simulink model "InverseDynamicsTest"  (R2021b)
settings: Solver=FixedStepAuto  StartTime=0.0  StopTime=5  FixedStep=Ts  RelTol=1e-3
values from neighbouring files (symbols this model uses):
  alphas_m = 25.0 * ones(1,dh.dof)    [setup_teleop.m]
  gravity = [0 0 9.81]'    [setup_robot.m]
  lambdas_m = 7.5 * ones(1,dh.dof)    [setup_teleop.m]
  zdq_A = [1 3*wc 3*wc^2 wc^3]    [setup_teleop.m]
  zdq_B = [0 0 0 wc^3]    [setup_teleop.m]
undefined symbols (not defined in the file or in its folder): conf, dh, x0
libraries: simulink x2, robotcorelib x1, vrlib x1
settings Model: Creator=eros  LastModifiedBy=Sebastiano
settings SolverCC: AlgebraicLoopSolver=TrustRegion
settings DebuggingCC: SFMachineParentedDataDiag=warning

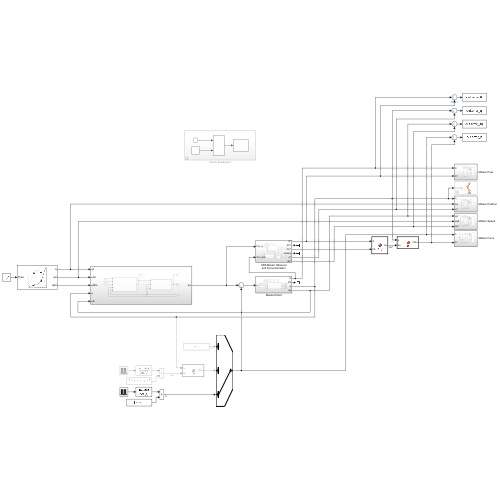
[thumbnail: Simulink's stored preview of the top-level diagram]
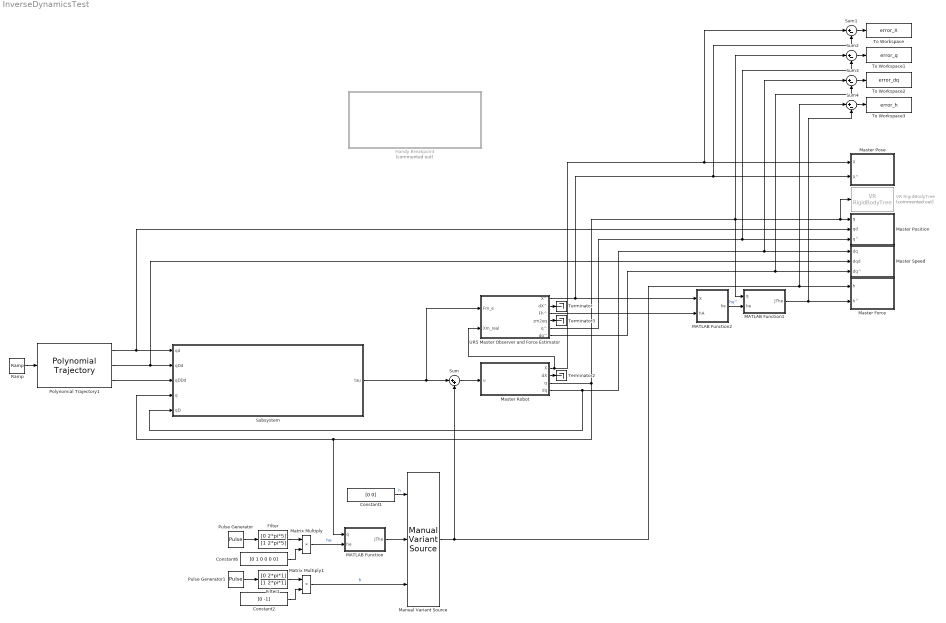
== system InverseDynamicsTest ==
  Constant1 : Constant  Value=[0 0]
  Constant2 : Constant  Value=[0 -1]
  Constant6 : Constant  Value=[0 1 0 0 0 0]
  Filter : TransferFcn  Numerator=[0 2*pi*5]  Denominator=[1 2*pi*5]
  Filter1 : TransferFcn  Numerator=[0 2*pi*1]  Denominator=[1 2*pi*1]
  Handy Breakpoint : Subsystem  Commented=on
  MATLAB Function : MATLAB Function  TreatAsAtomicUnit=on
  MATLAB Function1 : MATLAB Function  TreatAsAtomicUnit=on
  MATLAB Function2 : MATLAB Function  TreatAsAtomicUnit=on
  Manual Variant Source : simulink/Signal Routing/Manual Variant Source  NumChoices=3  LabelModeActiveChoice=V_3
  Master Force : Subsystem
  Master Pose : Subsystem
  Master Position : Subsystem
  Master Robot : Subsystem
  Master Speed : Subsystem
  Matrix Multiply : Product
  Matrix Multiply1 : Product
  Polynomial Trajectory1 : robotcorelib/Polynomial Trajectory  WaypointSource=Internal  Waypoints=[conf.init.q0 conf.init.q0]  TimePoints=[ 0, 5]  TimeInterval=[ 1, 4 ]  Method=Cubic Polynomial  ParameterSource=Internal  VelocityBoundaryCondition=zeros( dh.dof, 2 )  AccelerationBoundaryCondition=zeros( 2, 5 )  SimulateUsing=Code generation
  Pulse Generator : DiscretePulseGenerator  PulseType=Time based  Amplitude=25  Period=3  PulseWidth=50  PhaseDelay=0.5
  Pulse Generator1 : DiscretePulseGenerator  PulseType=Time based  Amplitude=25  Period=3  PulseWidth=50  PhaseDelay=0.5
  Ramp : simulink/Sources/Ramp  slope=1  start=0  InitialOutput=0
  Subsystem : Subsystem
  Sum : Sum  Inputs=|++
  Sum{1..4} (4 alike) : Sum  Inputs=|+-
  Terminator : Terminator
  Terminator2 : Terminator
  Terminator3 : Terminator
  To Workspace : ToWorkspace  VariableName=error_X  SaveFormat=Timeseries  SampleTime=-1
  To Workspace1 : ToWorkspace  VariableName=error_q  SaveFormat=Timeseries  SampleTime=-1
  To Workspace2 : ToWorkspace  VariableName=error_dq  SaveFormat=Timeseries  SampleTime=-1
  To Workspace3 : ToWorkspace  VariableName=error_h  SaveFormat=Timeseries  SampleTime=-1
  UR5 Master Observer and Force Estimator : Subsystem
  VR RigidBodyTree : vrlib/VR RigidBodyTree  Commented=on  RBT=UR5_robot  useRBT=off  Ts=0.02  ForceViewerOpen=off
      settings: SourceProductBaseCode=SL
  wires:
  Master Robot/4(dq) -> Sum3/1, Master Speed/1(dq), Subsystem/5(qD)
  Polynomial Trajectory1/1 -> Master Position/2(qd), Subsystem/1(qd)
  Polynomial Trajectory1/2 -> Master Speed/2(dqd), Subsystem/2(qDd)
  Ramp/1 -> Polynomial Trajectory1/1
  Sum/1 -> Master Robot/1(u)
  Manual Variant Source/1 -> Master Force/1(h), Sum4/1, Sum/2
  Pulse Generator/1 -> Filter/1
  Constant6/1 -> Matrix Multiply/2
  Matrix Multiply/1 -> MATLAB Function/2(he)  "he"
  Filter/1 -> Matrix Multiply/1
  UR5 Master Observer and Force Estimator/5(q^) -> Master Position/3(q^), Sum2/2
  UR5 Master Observer and Force Estimator/3(Fh^) -> MATLAB Function2/2(hA)
  UR5 Master Observer and Force Estimator/6(dq^) -> Master Speed/3(dq^), Sum3/2
  Master Robot/1(X) -> Master Pose/1(X), Sum1/1, UR5 Master Observer and Force Estimator/2(Xm_real)
  Master Robot/2(dX) -> Terminator2/1
  UR5 Master Observer and Force Estimator/4(zm2eq) -> Terminator3/1
  UR5 Master Observer and Force Estimator/2(dX^) -> Terminator/1
  UR5 Master Observer and Force Estimator/1(X^) -> Master Pose/2(X^), Sum1/2, MATLAB Function2/1(X)
  Constant1/1 -> Manual Variant Source/1  "h"
  MATLAB Function2/1(he) -> MATLAB Function1/2(he)  "he^"
  Master Robot/3(q) -> VR RigidBodyTree/1, Master Position/1(q), MATLAB Function1/1(q), Sum2/1, Subsystem/4(q), MATLAB Function/1(q)
  MATLAB Function1/1(JThe) -> Master Force/2(h^), Sum4/2
  MATLAB Function/1(JThe) -> Manual Variant Source/2
  Matrix Multiply1/1 -> Manual Variant Source/3  "h"
  Constant2/1 -> Matrix Multiply1/2
  Filter1/1 -> Matrix Multiply1/1
  Pulse Generator1/1 -> Filter1/1
  Sum1/1 -> To Workspace/1
  Sum2/1 -> To Workspace1/1
  Sum3/1 -> To Workspace2/1
  Sum4/1 -> To Workspace3/1
  Subsystem/1(tau) -> Sum/1, UR5 Master Observer and Force Estimator/1(Fm_e)
  Polynomial Trajectory1/3 -> Subsystem/3(qDDd)

== system InverseDynamicsTest/Handy Breakpoint ==
  Assertion : Assertion  AssertionFailFcn=set_param(bdroot,'SimulationCommand','pause')  StopWhenAssertionFail=off
  Clock : Clock
  Constant : Constant  Value=0.5
  Relational Operator : RelationalOperator  Operator=<  OutDataTypeStr=boolean  RndMeth=Simplest
  wires:
  Relational Operator/1 -> Assertion/1
  Constant/1 -> Relational Operator/2
  Clock/1 -> Relational Operator/1

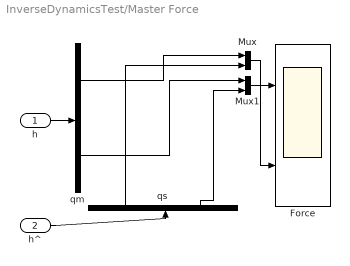
== system InverseDynamicsTest/Master Force ==
  h : Inport
  h^ : Inport  Port=2
  Force : Scope  NumInputPorts=2
  Mux : Mux  Inputs=2
  Mux1 : Mux  Inputs=2
  qm : Demux  Outputs=dh.dof
  qs : Demux  Outputs=dh.dof
  wires:
  h/1 -> qm/1
  h^/1 -> qs/1
  qm/1 -> Mux/1
  qs/1 -> Mux/2
  qm/2 -> Mux1/1
  qs/2 -> Mux1/2
  Mux/1 -> Force/1
  Mux1/1 -> Force/2

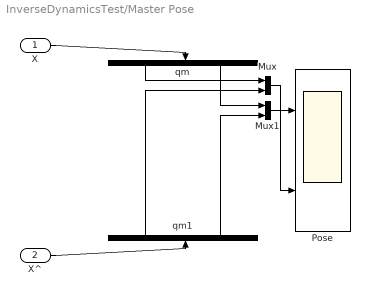
== system InverseDynamicsTest/Master Pose ==
  X : Inport
  X^ : Inport  Port=2
  Mux : Mux  Inputs=2
  Mux1 : Mux  Inputs=2
  Pose : Scope  NumInputPorts=2
  qm : Demux  Outputs=dh.dof
  qm1 : Demux  Outputs=dh.dof
  wires:
  X/1 -> qm/1
  qm/1 -> Mux/1
  qm/2 -> Mux1/1
  Mux/1 -> Pose/1
  Mux1/1 -> Pose/2
  qm1/2 -> Mux1/2
  X^/1 -> qm1/1
  qm1/1 -> Mux/2

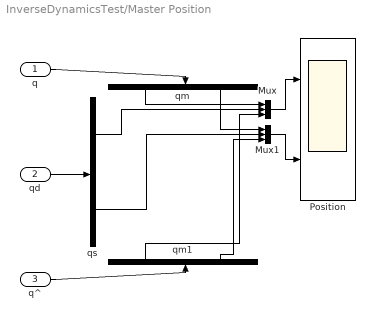
== system InverseDynamicsTest/Master Position ==
  q : Inport
  qd : Inport  Port=2
  q^ : Inport  Port=3
  Mux : Mux  Inputs=3
  Mux1 : Mux  Inputs=3
  Position : Scope  NumInputPorts=2
  qm : Demux  Outputs=dh.dof
  qm1 : Demux  Outputs=dh.dof
  qs : Demux  Outputs=dh.dof
  wires:
  q/1 -> qm/1
  qd/1 -> qs/1
  qm/1 -> Mux/1
  qs/1 -> Mux/2
  qm/2 -> Mux1/1
  qs/2 -> Mux1/2
  Mux/1 -> Position/1
  Mux1/1 -> Position/2
  qm1/2 -> Mux1/3
  q^/1 -> qm1/1
  qm1/1 -> Mux/3

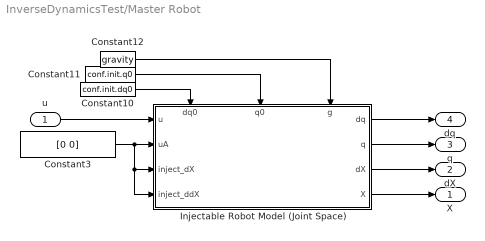
== system InverseDynamicsTest/Master Robot ==
  u : Inport
  Constant10 : Constant  Value=conf.init.dq0
  Constant11 : Constant  Value=conf.init.q0
  Constant12 : Constant  Value=gravity
  Constant3 : Constant  Value=[0 0]
  Injectable Robot Model (Joint Space) : Subsystem
      settings: PortSchema="{\"entries\":[{\"content\":{\"sides\":[{\"content\":{\"connectorIds\":[\"In1\",\"In2\",\"In3\",\"In4\"]},\"type\":\"ConnectorPlacement.EquallySpacedRectSide\",\"uuid\":\"a8701c64-329e-4144-b882-ecf5d621aff2\"},{\"content\":{\"connectorIds\":[\"Out1\",\"Out2\",\"Out3\",\"Out4\"],\"side\":\"RIGHT\"},\"type\":\"ConnectorPlacement.EquallySpacedRectSide\",\"uuid\":\"4e168703-1cb9-438c-bc6b-9b2d7fbb809e\"},{\"content\":{\"connectorIds\":[\"In5\",\"In6\",\"In7\"],\"side\":\"TOP\"},\"type\":\"ConnectorPlacement.EquallySpacedRectSide\",\"uuid\":\"8fbcb29e-7fab-4224-b4ad-ee01c13d675a\"}]},\"type\":\"ConnectorPlacement.EquallySpacedConnector\",\"uuid\":\"fa721fab-1ce6-4fdf-95fa-8ada3ed2d65c\"}],\"packageUris\":[\"http://schema.mathworks.com/mf0/Connector/R2020b\"],\"version\":\"1.0\"}"
  X : Outport
  dX : Outport  Port=2
  q : Outport  Port=3
  dq : Outport  Port=4
  wires:
  Constant10/1 -> Injectable Robot Model (Joint Space)/5(dq0)
  Constant3/1 -> Injectable Robot Model (Joint Space)/4(inject_ddX), Injectable Robot Model (Joint Space)/3(inject_dX), Injectable Robot Model (Joint Space)/2(uA)
  Constant11/1 -> Injectable Robot Model (Joint Space)/6(q0)
  Injectable Robot Model (Joint Space)/2(q) -> q/1
  Injectable Robot Model (Joint Space)/3(dX) -> dX/1
  Constant12/1 -> Injectable Robot Model (Joint Space)/7(g)
  Injectable Robot Model (Joint Space)/4(X) -> X/1
  Injectable Robot Model (Joint Space)/1(dq) -> dq/1
  u/1 -> Injectable Robot Model (Joint Space)/1(u)

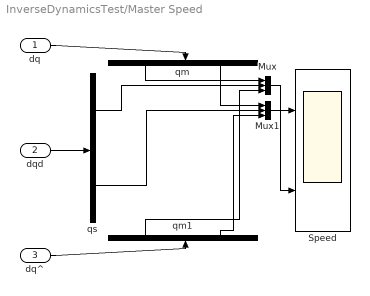
== system InverseDynamicsTest/Master Speed ==
  dq : Inport
  dqd : Inport  Port=2
  dq^ : Inport  Port=3
  Mux : Mux  Inputs=3
  Mux1 : Mux  Inputs=3
  Speed : Scope  NumInputPorts=2
  qm : Demux  Outputs=dh.dof
  qm1 : Demux  Outputs=dh.dof
  qs : Demux  Outputs=dh.dof
  wires:
  dq/1 -> qm/1
  dqd/1 -> qs/1
  qm/1 -> Mux/1
  qs/1 -> Mux/2
  qm/2 -> Mux1/1
  qs/2 -> Mux1/2
  Mux/1 -> Speed/1
  Mux1/1 -> Speed/2
  qm1/2 -> Mux1/3
  dq^/1 -> qm1/1
  qm1/1 -> Mux/3

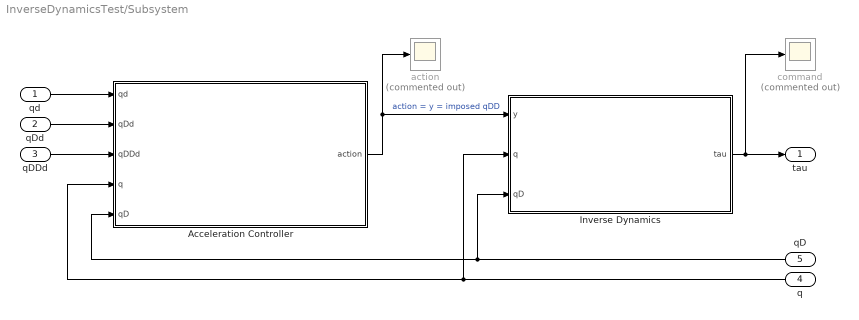
== system InverseDynamicsTest/Subsystem ==
  qd : Inport
  qDd : Inport  Port=2
  qDDd : Inport  Port=3
  q : Inport  Port=4
  qD : Inport  Port=5
  Acceleration Controller : Subsystem
  Inverse Dynamics : Subsystem
  action : Scope  Commented=on
  command : Scope  Commented=on
  tau : Outport
  wires:
  qD/1 -> Acceleration Controller/5(qD), Inverse Dynamics/3(qD)
  qd/1 -> Acceleration Controller/1(qd)
  q/1 -> Inverse Dynamics/2(q), Acceleration Controller/4(q)
  Inverse Dynamics/1(tau) -> tau/1, command/1
  qDDd/1 -> Acceleration Controller/3(qDDd)
  qDd/1 -> Acceleration Controller/2(qDd)
  Acceleration Controller/1(action) -> Inverse Dynamics/1(y), action/1  "action = y = imposed qDD"

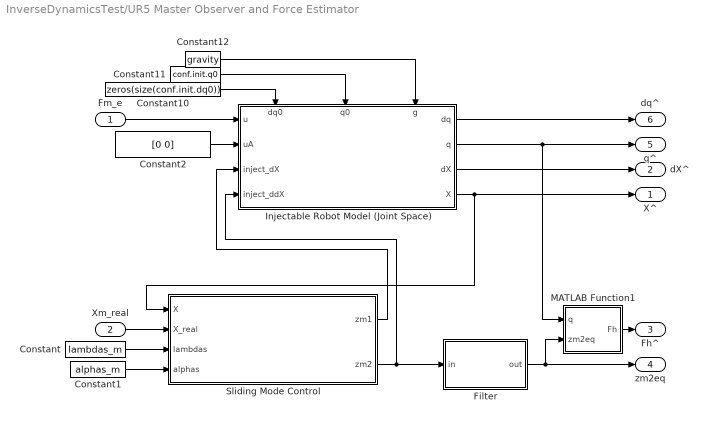
== system InverseDynamicsTest/UR5 Master Observer and Force Estimator ==
  Fm_e : Inport
  Xm_real : Inport  Port=2
  Constant : Constant  Value=lambdas_m
  Constant1 : Constant  Value=alphas_m
  Constant10 : Constant  Value=zeros(size(conf.init.dq0))
  Constant11 : Constant  Value=conf.init.q0
  Constant12 : Constant  Value=gravity
  Constant2 : Constant  Value=[0 0]
  Filter : Subsystem
  Injectable Robot Model (Joint Space) : Subsystem
      settings: PortSchema="{\"entries\":[{\"content\":{\"sides\":[{\"content\":{\"connectorIds\":[\"In1\",\"In2\",\"In3\",\"In4\"]},\"type\":\"ConnectorPlacement.EquallySpacedRectSide\",\"uuid\":\"a8701c64-329e-4144-b882-ecf5d621aff2\"},{\"content\":{\"connectorIds\":[\"Out1\",\"Out2\",\"Out3\",\"Out4\"],\"side\":\"RIGHT\"},\"type\":\"ConnectorPlacement.EquallySpacedRectSide\",\"uuid\":\"4e168703-1cb9-438c-bc6b-9b2d7fbb809e\"},{\"content\":{\"connectorIds\":[\"In5\",\"In6\",\"In7\"],\"side\":\"TOP\"},\"type\":\"ConnectorPlacement.EquallySpacedRectSide\",\"uuid\":\"8fbcb29e-7fab-4224-b4ad-ee01c13d675a\"}]},\"type\":\"ConnectorPlacement.EquallySpacedConnector\",\"uuid\":\"fa721fab-1ce6-4fdf-95fa-8ada3ed2d65c\"}],\"packageUris\":[\"http://schema.mathworks.com/mf0/Connector/R2020b\"],\"version\":\"1.0\"}"
  MATLAB Function1 : MATLAB Function  TreatAsAtomicUnit=on
  Sliding Mode Control : Subsystem
  X^ : Outport
  dX^ : Outport  Port=2
  Fh^ : Outport  Port=3
  zm2eq : Outport  Port=4
  q^ : Outport  Port=5
  dq^ : Outport  Port=6
  wires:
  Filter/1(out) -> MATLAB Function1/2(zm2eq), zm2eq/1
  Sliding Mode Control/1(zm1) -> Injectable Robot Model (Joint Space)/3(inject_dX)
  Sliding Mode Control/2(zm2) -> Injectable Robot Model (Joint Space)/4(inject_ddX), Filter/1(in)
  Constant1/1 -> Sliding Mode Control/4(alphas)
  Constant/1 -> Sliding Mode Control/3(lambdas)
  Xm_real/1 -> Sliding Mode Control/2(X_real)
  Injectable Robot Model (Joint Space)/4(X) -> X^/1, Sliding Mode Control/1(X)
  Injectable Robot Model (Joint Space)/3(dX) -> dX^/1
  Constant11/1 -> Injectable Robot Model (Joint Space)/6(q0)
  Fm_e/1 -> Injectable Robot Model (Joint Space)/1(u)
  Constant10/1 -> Injectable Robot Model (Joint Space)/5(dq0)
  Injectable Robot Model (Joint Space)/1(dq) -> dq^/1
  Constant12/1 -> Injectable Robot Model (Joint Space)/7(g)
  Injectable Robot Model (Joint Space)/2(q) -> MATLAB Function1/1(q), q^/1
  MATLAB Function1/1(Fh) -> Fh^/1
  Constant2/1 -> Injectable Robot Model (Joint Space)/2(uA)

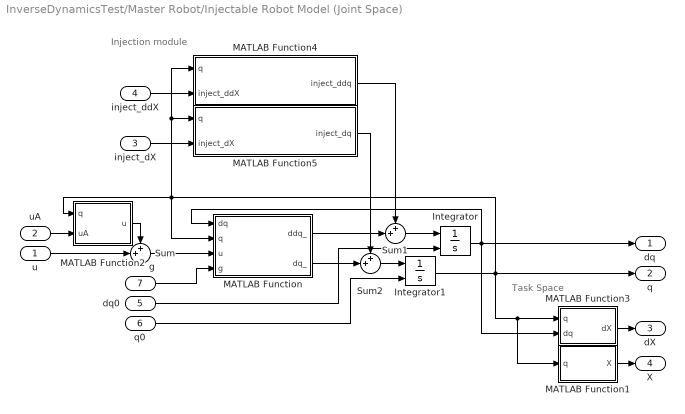
== system InverseDynamicsTest/Master Robot/Injectable Robot Model (Joint Space) ==
  note: Injection module
  note: Task Space
  u : Inport
  uA : Inport  Port=2
  inject_dX : Inport  Port=3
  inject_ddX : Inport  Port=4
  dq0 : Inport  Port=5
  q0 : Inport  Port=6
  g : Inport  Port=7
  Integrator : Integrator  InitialConditionSource=external  InitialCondition=x0
  Integrator1 : Integrator  InitialConditionSource=external  InitialCondition=x0
  MATLAB Function : MATLAB Function  TreatAsAtomicUnit=on
  MATLAB Function1 : MATLAB Function  TreatAsAtomicUnit=on
  MATLAB Function2 : MATLAB Function  TreatAsAtomicUnit=on
  MATLAB Function3 : MATLAB Function  TreatAsAtomicUnit=on
  MATLAB Function4 : MATLAB Function  TreatAsAtomicUnit=on
  MATLAB Function5 : MATLAB Function  TreatAsAtomicUnit=on
  Sum : Sum  Inputs=++|
  Sum1 : Sum  Inputs=++|
  Sum2 : Sum  Inputs=++|
  dq : Outport
  q : Outport  Port=2
  dX : Outport  Port=3
  X : Outport  Port=4
  wires:
  g/1 -> MATLAB Function/4(g)
  u/1 -> Sum/2
  dq0/1 -> Integrator/2
  Integrator1/1 -> q/1, MATLAB Function1/1(q), MATLAB Function3/1(q), MATLAB Function/2(q), MATLAB Function4/1(q), MATLAB Function5/1(q), MATLAB Function2/1(q)
  uA/1 -> MATLAB Function2/2(uA)
  MATLAB Function1/1(X) -> X/1
  Integrator/1 -> dq/1, MATLAB Function3/2(dq), MATLAB Function/1(dq)
  MATLAB Function3/1(dX) -> dX/1
  MATLAB Function2/1(u) -> Sum/1
  Sum/1 -> MATLAB Function/3(u)
  MATLAB Function/1(ddq_) -> Sum1/2
  q0/1 -> Integrator1/2
  Sum1/1 -> Integrator/1
  MATLAB Function/2(dq_) -> Sum2/2
  Sum2/1 -> Integrator1/1
  inject_ddX/1 -> MATLAB Function4/2(inject_ddX)
  inject_dX/1 -> MATLAB Function5/2(inject_dX)
  MATLAB Function4/1(inject_ddq) -> Sum1/1
  MATLAB Function5/1(inject_dq) -> Sum2/1

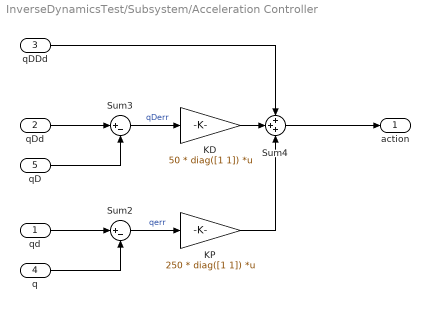
== system InverseDynamicsTest/Subsystem/Acceleration Controller ==
  qd : Inport
  qDd : Inport  Port=2
  qDDd : Inport  Port=3
  q : Inport  Port=4
  qD : Inport  Port=5
  KD : Gain  Gain=50 * diag([1 1])  Multiplication=Matrix(K*u) (u vector)
  KP : Gain  Gain=250 * diag([1 1])  Multiplication=Matrix(K*u) (u vector)
  Sum2 : Sum  Inputs=|+-
  Sum3 : Sum  Inputs=|+-
  Sum4 : Sum  Inputs=+++
  action : Outport
  wires:
  qDd/1 -> Sum3/1
  KD/1 -> Sum4/2
  KP/1 -> Sum4/3
  qD/1 -> Sum3/2
  Sum3/1 -> KD/1  "qDerr"
  Sum4/1 -> action/1
  Sum2/1 -> KP/1  "qerr"
  qd/1 -> Sum2/1
  qDDd/1 -> Sum4/1
  q/1 -> Sum2/2

== system InverseDynamicsTest/Subsystem/Inverse Dynamics ==
  y : Inport
  q : Inport  Port=2
  qD : Inport  Port=3
  MATLAB Function : MATLAB Function  TreatAsAtomicUnit=on
  MATLAB Function1 : MATLAB Function  TreatAsAtomicUnit=on
  Sum1 : Sum  Inputs=++|
  tau : Outport
  wires:
  qD/1 -> MATLAB Function/2(qD)
  MATLAB Function/1(n) -> Sum1/1
  MATLAB Function1/1(taud) -> Sum1/2
  q/1 -> MATLAB Function1/1(q), MATLAB Function/1(q)
  y/1 -> MATLAB Function1/2(y)
  Sum1/1 -> tau/1  "tau"

== system InverseDynamicsTest/UR5 Master Observer and Force Estimator/Filter ==
  in : Inport
  Demux : Demux  Outputs=2
  Filter : TransferFcn  Numerator=zdq_B  Denominator=zdq_A
  Filter1 : TransferFcn  Numerator=zdq_B  Denominator=zdq_A
  Mux : Mux  Inputs=2
  out : Outport
  wires:
  Demux/2 -> Filter1/1
  Demux/1 -> Filter/1
  in/1 -> Demux/1
  Mux/1 -> out/1
  Filter/1 -> Mux/1
  Filter1/1 -> Mux/2

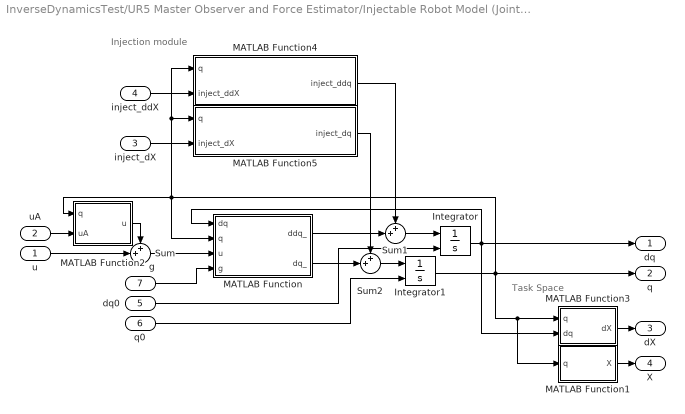
== system InverseDynamicsTest/UR5 Master Observer and Force Estimator/Injectable Robot Model (Joint Space) ==
  note: Injection module
  note: Task Space
  u : Inport
  uA : Inport  Port=2
  inject_dX : Inport  Port=3
  inject_ddX : Inport  Port=4
  dq0 : Inport  Port=5
  q0 : Inport  Port=6
  g : Inport  Port=7
  Integrator : Integrator  InitialConditionSource=external  InitialCondition=x0
  Integrator1 : Integrator  InitialConditionSource=external  InitialCondition=x0
  MATLAB Function : MATLAB Function  TreatAsAtomicUnit=on
  MATLAB Function1 : MATLAB Function  TreatAsAtomicUnit=on
  MATLAB Function2 : MATLAB Function  TreatAsAtomicUnit=on
  MATLAB Function3 : MATLAB Function  TreatAsAtomicUnit=on
  MATLAB Function4 : MATLAB Function  TreatAsAtomicUnit=on
  MATLAB Function5 : MATLAB Function  TreatAsAtomicUnit=on
  Sum : Sum  Inputs=++|
  Sum1 : Sum  Inputs=++|
  Sum2 : Sum  Inputs=++|
  dq : Outport
  q : Outport  Port=2
  dX : Outport  Port=3
  X : Outport  Port=4
  wires:
  g/1 -> MATLAB Function/4(g)
  u/1 -> Sum/2
  dq0/1 -> Integrator/2
  Integrator1/1 -> q/1, MATLAB Function1/1(q), MATLAB Function3/1(q), MATLAB Function/2(q), MATLAB Function4/1(q), MATLAB Function5/1(q), MATLAB Function2/1(q)
  uA/1 -> MATLAB Function2/2(uA)
  MATLAB Function1/1(X) -> X/1
  Integrator/1 -> dq/1, MATLAB Function3/2(dq), MATLAB Function/1(dq)
  MATLAB Function3/1(dX) -> dX/1
  MATLAB Function2/1(u) -> Sum/1
  Sum/1 -> MATLAB Function/3(u)
  MATLAB Function/1(ddq_) -> Sum1/2
  q0/1 -> Integrator1/2
  Sum1/1 -> Integrator/1
  MATLAB Function/2(dq_) -> Sum2/2
  Sum2/1 -> Integrator1/1
  inject_ddX/1 -> MATLAB Function4/2(inject_ddX)
  inject_dX/1 -> MATLAB Function5/2(inject_dX)
  MATLAB Function4/1(inject_ddq) -> Sum1/1
  MATLAB Function5/1(inject_dq) -> Sum2/1

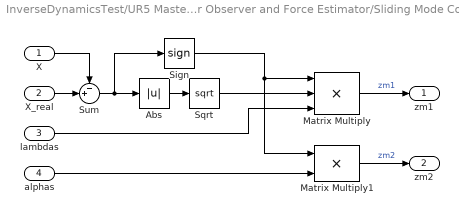
== system InverseDynamicsTest/UR5 Master Observer and Force Estimator/Sliding Mode Control ==
  X : Inport
  X_real : Inport  Port=2
  lambdas : Inport  Port=3
  alphas : Inport  Port=4
  Abs : Abs
  Matrix Multiply : Product  Inputs=***
  Matrix Multiply1 : Product
  Sign : Signum
  Sqrt : Sqrt  SaturateOnIntegerOverflow=on
  Sum : Sum  Inputs=-+|
  zm1 : Outport
  zm2 : Outport  Port=2
  wires:
  Sum/1 -> Sign/1, Abs/1
  Abs/1 -> Sqrt/1
  X/1 -> Sum/1
  lambdas/1 -> Matrix Multiply/3
  Sqrt/1 -> Matrix Multiply/2
  X_real/1 -> Sum/2
  Matrix Multiply/1 -> zm1/1  "zm1"
  Matrix Multiply1/1 -> zm2/1  "zm2"
  alphas/1 -> Matrix Multiply1/2
  Sign/1 -> Matrix Multiply/1, Matrix Multiply1/1

== matlab function InverseDynamicsTest/Subsystem/Inverse Dynamics/MATLAB Function ==
  data: q input; qD input; n output; dh parameter; gravity parameter
function n = n(q, qD, dh, gravity)

    C = C_rne(dh, q, qD);
    G = G_rne(dh, q, gravity);

    n = C * qD + G;

== matlab function InverseDynamicsTest/Master Robot/Injectable Robot Model (Joint Space)/MATLAB Function5 ==
  data: q input size=dh.dof; inject_dq output size=dh.dof; inject_dX input size=2; dh parameter
function inject_dq = get_inject_dq(q, inject_dX, dh)
    JA = JA_rne(dh, q);
    inject_dq = pinv(JA) * inject_dX;
end

== matlab function InverseDynamicsTest/Subsystem/Inverse Dynamics/MATLAB Function1 ==
  data: q input; taud output; y input; dh parameter
function taud = B(q, y, dh)

    B = B_rne(dh, q);

    taud = B*y;

== matlab function InverseDynamicsTest/UR5 Master Observer and Force Estimator/Injectable Robot Model (Joint Space)/MATLAB Function1 ==
  data: X output; q input; dh parameter
function X = K(q, dh)
    X = K_rne(dh, q);
end

== matlab function InverseDynamicsTest/MATLAB Function ==
  data: JThe output; q input; he input; dh parameter
function JThe = JT(q, he, dh)
    JThe = J_rne(dh, q)' * he;
end

== matlab function InverseDynamicsTest/UR5 Master Observer and Force Estimator/Injectable Robot Model (Joint Space)/MATLAB Function3 ==
  data: dh parameter; dX output; q input; dq input
function dX = JA(dh, q, dq)
    dX = JA_rne(dh, q)*dq;
end

== matlab function InverseDynamicsTest/UR5 Master Observer and Force Estimator/Injectable Robot Model (Joint Space)/MATLAB Function4 ==
  data: q input size=dh.dof; inject_ddq output size=dh.dof; inject_ddX input size=2; dh parameter
function inject_ddq = get_inject_ddq(q, inject_ddX, dh)
    JA = JA_rne(dh, q);
    inject_ddq = pinv(JA) * inject_ddX;
end

== matlab function InverseDynamicsTest/MATLAB Function1 ==
  data: JThe output; q input; he input; dh parameter
function JThe = JT(q, he, dh)
    JThe = J_rne(dh, q)' * he;
end

== matlab function InverseDynamicsTest/UR5 Master Observer and Force Estimator/Injectable Robot Model (Joint Space)/MATLAB Function5 ==
  data: q input size=dh.dof; inject_dq output size=dh.dof; inject_dX input size=2; dh parameter
function inject_dq = get_inject_dq(q, inject_dX, dh)
    JA = JA_rne(dh, q);
    inject_dq = pinv(JA) * inject_dX;
end

== matlab function InverseDynamicsTest/Master Robot/Injectable Robot Model (Joint Space)/MATLAB Function ==
  data ddq_ settings: updateMethod=SF_CONTINUOUS_TIME_DATA
  data dq_ settings: updateMethod=SF_CONTINUOUS_TIME_DATA
  data dq settings: updateMethod=SF_CONTINUOUS_TIME_DATA
  data q settings: updateMethod=SF_CONTINUOUS_TIME_DATA
  data u settings: updateMethod=SF_CONTINUOUS_TIME_DATA
  data: ddq_ output size=dh.dof; dq_ output size=dh.dof; dq input size=dh.dof; q input size=dh.dof; u input size=dh.dof; g input size=3; dh parameter
function [ddq_, dq_]  = RobotSystem(dq, q, u, g, dh)
    
    % compute dynamics
    B = B_rne(dh, q);
    C = C_rne(dh, q, dq);
    G = G_rne(dh, q, g);

    dq_ = dq(1:dh.dof);

    ddq = B \ (u - C*dq - G);
    ddq_ = ddq(1:dh.dof);
end

== matlab function InverseDynamicsTest/Master Robot/Injectable Robot Model (Joint Space)/MATLAB Function1 ==
  data: X output; q input; dh parameter
function X = K(q, dh)
    X = K_rne(dh, q);
end

== matlab function InverseDynamicsTest/UR5 Master Observer and Force Estimator/Injectable Robot Model (Joint Space)/MATLAB Function2 ==
  data: q input; uA input; u output; dh parameter
function u = JAT(q,uA, dh)
    u = JA_rne(dh,q)' * uA;
end

== matlab function InverseDynamicsTest/MATLAB Function2 ==
  data: he output; X input; hA input
function he = TAT_1(X, hA)
    TA_ = TA(X);
    rpinv = (TA_*TA_') \ TA_;
    he = rpinv * hA;
end

== matlab function InverseDynamicsTest/Master Robot/Injectable Robot Model (Joint Space)/MATLAB Function2 ==
  data: q input; uA input; u output; dh parameter
function u = JAT(q,uA, dh)
    u = JA_rne(dh,q)' * uA;
end

== matlab function InverseDynamicsTest/Master Robot/Injectable Robot Model (Joint Space)/MATLAB Function3 ==
  data: dh parameter; dX output; q input; dq input
function dX = JA(dh, q, dq)
    dX = JA_rne(dh, q)*dq;
end

== matlab function InverseDynamicsTest/UR5 Master Observer and Force Estimator/MATLAB Function1 ==
  data: Fh output; q input; zm2eq input; dh parameter
function Fh = BA_zm(q, zm2eq, dh)
     BA = BA_rne(dh, q);
     Fh = BA * zm2eq;
end

== matlab function InverseDynamicsTest/Master Robot/Injectable Robot Model (Joint Space)/MATLAB Function4 ==
  data: q input size=dh.dof; inject_ddq output size=dh.dof; inject_ddX input size=2; dh parameter
function inject_ddq = get_inject_ddq(q, inject_ddX, dh)
    JA = JA_rne(dh, q);
    inject_ddq = pinv(JA) * inject_ddX;
end

== matlab function InverseDynamicsTest/UR5 Master Observer and Force Estimator/Injectable Robot Model (Joint Space)/MATLAB Function ==
  data ddq_ settings: updateMethod=SF_CONTINUOUS_TIME_DATA
  data dq_ settings: updateMethod=SF_CONTINUOUS_TIME_DATA
  data dq settings: updateMethod=SF_CONTINUOUS_TIME_DATA
  data q settings: updateMethod=SF_CONTINUOUS_TIME_DATA
  data u settings: updateMethod=SF_CONTINUOUS_TIME_DATA
  data: ddq_ output size=dh.dof; dq_ output size=dh.dof; dq input size=dh.dof; q input size=dh.dof; u input size=dh.dof; g input size=3; dh parameter
function [ddq_, dq_]  = RobotSystem(dq, q, u, g, dh)
    
    % compute dynamics
    B = B_rne(dh, q);
    C = C_rne(dh, q, dq);
    G = G_rne(dh, q, g);

    dq_ = dq(1:dh.dof);

    ddq = B \ (u - C*dq - G);
    ddq_ = ddq(1:dh.dof);
end
